simulink model "target_generation_test"  (R2016b)
settings: Solver=VariableStepAuto  StartTime=0.0  StopTime=1  RelTol=1e-3
values from neighbouring files (symbols this model uses):
  sc2gs_eci_unit = zeros(3,1)    [target_generation_test_init.m]
  sc2sun_eci_unit = [0.5670; 0.3732; -0.7343]    [target_generation_test_init.m]
  sc_mode = 31    [target_generation_test_init.m]
  vel_eci_kmps = [0.9082; 0.3185; 0.2715]    [target_generation_test_init.m]
undefined symbols (not defined in the file or in its folder): target_generation_lib
libraries: aerolibtransform2 x1
settings Model: Creator=Taylor  LastModifiedBy=taylorreynolds

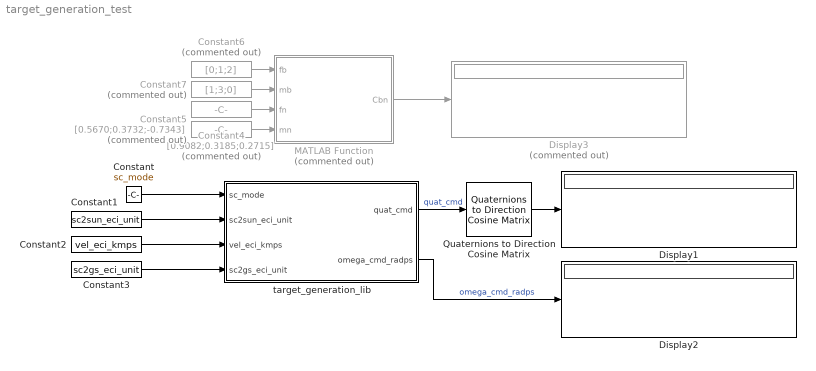
== system target_generation_test ==
  Constant : Constant  Value=sc_mode
  Constant1 : Constant  Value=sc2sun_eci_unit
  Constant2 : Constant  Value=vel_eci_kmps
  Constant3 : Constant  Value=sc2gs_eci_unit
  Constant4 : Constant  Commented=on  Value=[0.9082;0.3185;0.2715]
  Constant5 : Constant  Commented=on  Value=[0.5670;0.3732;-0.7343]
  Constant6 : Constant  Commented=on  Value=[0;1;2]
  Constant7 : Constant  Commented=on  Value=[1;3;0]
  Display1 : Display
  Display2 : Display
  Display3 : Display  Commented=on
  MATLAB Function : MATLAB Function  Commented=on  TreatAsAtomicUnit=on
  Quaternions to Direction Cosine Matrix : aerolibtransform2/Quaternions to  Direction Cosine Matrix
  target_generation_lib : Subsystem  AncestorBlock=target_generation_lib/target_generation_lib
  wires:
  Constant/1 -> target_generation_lib/1(sc_mode)
  Constant3/1 -> target_generation_lib/4(sc2gs_eci_unit)
  Constant2/1 -> target_generation_lib/3(vel_eci_kmps)
  Constant1/1 -> target_generation_lib/2(sc2sun_eci_unit)
  target_generation_lib/1(quat_cmd) -> Quaternions to Direction Cosine Matrix/1  "quat_cmd"
  Quaternions to Direction Cosine Matrix/1 -> Display1/1
  MATLAB Function/1(Cbn) -> Display3/1
  Constant7/1 -> MATLAB Function/2(mb)
  Constant6/1 -> MATLAB Function/1(fb)
  Constant5/1 -> MATLAB Function/4(mn)
  Constant4/1 -> MATLAB Function/3(fn)
  target_generation_lib/2(omega_cmd_radps) -> Display2/1  "omega_cmd_radps"

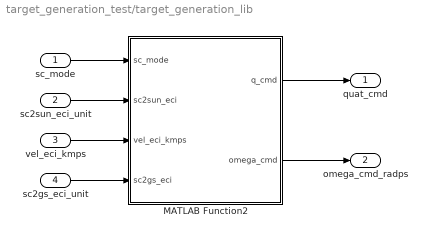
== system target_generation_test/target_generation_lib ==
  sc_mode : Inport
  sc2sun_eci_unit : Inport  Port=2
  vel_eci_kmps : Inport  Port=3
  sc2gs_eci_unit : Inport  Port=4
  MATLAB Function2 : MATLAB Function  TreatAsAtomicUnit=on
  quat_cmd : Outport
  omega_cmd_radps : Outport  Port=2
  wires:
  sc_mode/1 -> MATLAB Function2/1(sc_mode)
  sc2sun_eci_unit/1 -> MATLAB Function2/2(sc2sun_eci)
  vel_eci_kmps/1 -> MATLAB Function2/3(vel_eci_kmps)
  sc2gs_eci_unit/1 -> MATLAB Function2/4(sc2gs_eci)
  MATLAB Function2/1(q_cmd) -> quat_cmd/1
  MATLAB Function2/2(omega_cmd) -> omega_cmd_radps/1

== matlab function target_generation_test/target_generation_lib/MATLAB Function2 ==
  data: sc_mode input; q_cmd output; sc2sun_eci input; vel_eci_kmps input; sc2gs_eci input; omega_cmd output
function [q_cmd,omega_cmd]  = TRIAD(sc_mode,sc2sun_eci,vel_eci_kmps,sc2gs_eci)
%#codegen
% FSW Target Generation Library
%   UW HuskySat-1, ADCS Team
%   Last Updated: T. Reynolds 1.15.18

% Computes desired quaternion and angular velocity depending on the sc_mode
%   mode_logic.bdot             = 1;
%   mode_logic.desat_eclipse    = 2;
%   mode_logic.point            = 3;
%       point.velocity          = 31;
%       point.ground            = 32;
%       point.MPC               = 33;
%   mode_logic.low_power        = 4;

COM2    = [0; -1; 0];
PPT     = [0; 0; -1];
% PPT     = [0;1;2]; % these are used for testing only
% SP      = [1;3;0];

Cx5  = [ 1 0 0; 0 cosd(5) sind(5); 0 -sind(5) cosd(5)];


if( sc_mode == 31 )
    
     SP  = [0; 1; 0];
    
    % Body
    B1  = PPT./norm(PPT);
    B2  = SP./norm(SP);
    Xtb     = B1;
    Ytb     = cross(B1,B2)/norm(cross(B1,B2));
    Ztb     = cross(B1,cross(B1,B2))/norm(cross(B1,B2));
    
    % Inertial
    S1  = vel_eci_kmps./norm(vel_eci_kmps);
    S2  = sc2sun_eci./norm(sc2sun_eci);
    Xti     = S1;
    Yti     = cross(S1,S2)/norm(cross(S1,S2));
    Zti     = cross(S1,cross(S1,S2))/norm(cross(S1,S2));
    
    % Stack vectors
    Cb  = [Xtb, Ytb, Ztb];
    Ci  = [Xti, Yti, Zti];
    
    % Commanded DCM ( body to inertial )
    C_cmd   = Ci*Cb';
    % Commanded Angular Velocity
    omega_cmd   = [0;0;0]; % fill this in with mean motion
        
elseif( sc_mode == 32 )
    
    % Tilted so doesn't aling with COM2 -- chose a 5[deg] roll.
    SP      = Cx5*[0;1;0]; 
    
    % Body
    B1  = COM2./norm(COM2);
    B2  = SP./norm(SP);
    Xtb     = B1;
    Ytb     = cross(B1,B2)/norm(cross(B1,B2));
    Ztb     = cross(B1,cross(B1,B2))/norm(cross(B1,B2));
    
    % Inertial
    S1  = sc2gs_eci./norm(sc2gs_eci);
    S2  = sc2sun_eci./norm(sc2sun_eci);
    Xti     = S1;
    Yti     = cross(S1,S2)/norm(cross(S1,S2));
    Zti     = cross(S1,cross(S1,S2))/norm(cross(S1,S2));
    
    % Stack vectors
    Cb  = [Xtb, Ytb, Ztb];
    Ci  = [Xti, Yti, Zti];
    
    % Commanded DCM ( body to inertial )
    C_cmd   = Ci*Cb';
    % Commanded Angular Velocity
    omega_cmd   = [0;0;0]; % fill this in with mean motion
    
else
    C_cmd   = eye(3);
    omega_cmd   = zeros(3,1);
end

% Compute commanded quaternion from DCM
q_cmd   = myDCM2quat( C_cmd );

end


function q = DCM2quat( dcm )
    q   = zeros(4,1);
    
    tr = trace(dcm);

    if (tr > 0)
        sqtrp1 = sqrt( tr + 1.0 );
        
        q(1) = 0.5*sqtrp1; 
        q(2) = (dcm(2, 3) - dcm(3, 2))/(2.0*sqtrp1);
        q(3) = (dcm(3, 1) - dcm(1, 3))/(2.0*sqtrp1); 
        q(4) = (dcm(1, 2) - dcm(2, 1))/(2.0*sqtrp1); 
    else
        d = diag(dcm);
        if ((d(2) > d(1)) && (d(2) > d(3)))
            % max value at dcm(2,2)
            sqdip1 = sqrt(d(2) - d(1) - d(3) + 1.0 );
            
            q(3) = 0.5*sqdip1; 
            
            if ( sqdip1 ~= 0 )
                sqdip1 = 0.5/sqdip1;
            end
            
            q(1) = (dcm(3, 1) - dcm(1, 3))*sqdip1; 
            q(2) = (dcm(1, 2) + dcm(2, 1))*sqdip1; 
            q(4) = (dcm(2, 3) + dcm(3, 2))*sqdip1; 
        elseif (d(3) > d(1))
            % max value at dcm(3,3)
            sqdip1 = sqrt(d(3) - d(1) - d(2) + 1.0 );
            
            q(4) = 0.5*sqdip1; 
            
            if ( sqdip1 ~= 0 )
                sqdip1 = 0.5/sqdip1;
            end
            
            q(1) = (dcm(1, 2) - dcm(2, 1))*sqdip1;
            q(2) = (dcm(3, 1) + dcm(1, 3))*sqdip1; 
            q(3) = (dcm(2, 3) + dcm(3, 2))*sqdip1; 
        else
            % max value at dcm(1,1)
            sqdip1 = sqrt(d(1) - d(2) - d(3) + 1.0 );
            
            q(2) = 0.5*sqdip1; 
            
            if ( sqdip1 ~= 0 )
                sqdip1 = 0.5/sqdip1;
            end
            
            q(1) = (dcm(2, 3) - dcm(3, 2))*sqdip1; 
            q(3) = (dcm(1, 2) + dcm(2, 1))*sqdip1; 
            q(4) = (dcm(3, 1) + dcm(1, 3))*sqdip1; 
        end

    end

end

function q = myDCM2quat( DCM )

q   = zeros(4,1);

tr  = trace(DCM);

q(1)    = 0.5*sqrt(tr + 1);

if( q(1) ~= 0 )
    eta     = 1/(4*q(1));
    q(2)    = eta*(DCM(2,3) - DCM(3,2));
    q(3)    = eta*(DCM(3,1) - DCM(1,3));
    q(4)    = eta*(DCM(1,2) - DCM(2,1));
else
    q(2)  = sqrt(0.5*(DCM(1,1) + 1));
    q(3)  = sign(DCM(1,2))*sqrt(0.5*(DCM(2,2) + 1));
    q(4)  = sign(DCM(1,3))*sqrt(0.5*(DCM(3,3) + 1));
end


end

== matlab function target_generation_test/MATLAB Function ==
  data: fb input; Cbn output; mb input; fn input; mn input
function Cbn = TRIAD(fb, mb, fn, mn)
% Cbn = TRIAD(fb, mb, fn, mn)
% Function implements  TRIAD algorithm using measurements
% from three-component accelerometer with orthogonal axes and vector
% magnetometer
%
%   Input arguments:
%   fb  - Acceleration vector in body frame [3x1]
%   mb  - Magnetic field vector in body frame [3x1]
%   fn  - Gravity vector in navigation frame [3x1]
%   mn  - Magetic field vector in navigation frame [3x1]
%
%   Output arguments:
%   Cbn - estimated Direction Cosines Matrix (DCM)

W1 = fb/norm(fb);
W2 = mb/norm(mb);

V1 = fn;
V2 = mn;

Ou1 = W1;
Ou2 = cross(W1,W2)/norm(cross(W1,W2));
Ou3 = cross(W1,cross(W1,W2))/norm(cross(W1,W2));

R1 = V1;
R2 = cross(V1,V2)/norm(cross(V1,V2));
R3 = cross(V1,cross(V1,V2))/norm(cross(V1,V2));

Mou = [Ou1, Ou2, Ou3];
Mr = [R1, R2, R3];

%TRIAD DCM
Cbn = Mr*Mou';

end
